simulink model "gm_Fixed"  (R2022a)
settings: Solver=FixedStepDiscrete  StartTime=0.0  StopTime=10.0  RelTol=1e-3  EnableMultiTasking=on
InitFcn:
  | test_init
settings Model: Creator=highi  LastModifiedBy=highi
settings OptimizationCC: BlockReduction=off  ConditionallyExecuteInputs=off
settings DebuggingCC: InheritedTsInSrcMsg=none
settings HardwareCC: ProdBitPerPointer=32  ProdBitPerSizeT=32  ProdBitPerPtrDiffT=32  ProdLargestAtomicFloat=None  ProdIntDivRoundTo=Undefined  ProdEndianess=Unspecified  ProdWordSize=32  ProdHWDeviceType=ASIC/FPGA->ASIC/FPGA  TargetBitPerPointer=64  TargetBitPerSizeT=64  TargetBitPerPtrDiffT=64  TargetLongLongMode=on  TargetIntDivRoundTo=Zero  TargetEndianess=LittleEndian  TargetWordSize=64  TargetHWDeviceType=Custom Processor->MATLAB Host Computer  ProdEqTarget=off

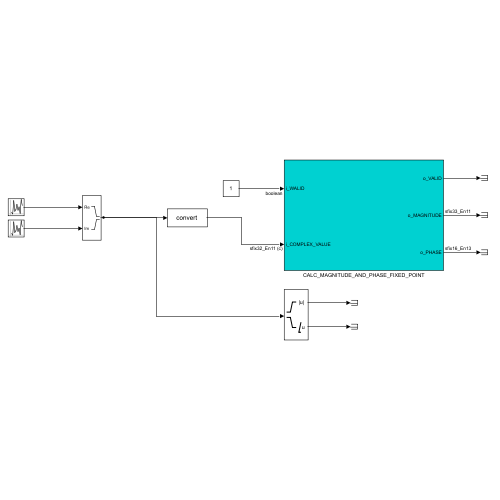
[thumbnail: Simulink's stored preview of the top-level diagram]
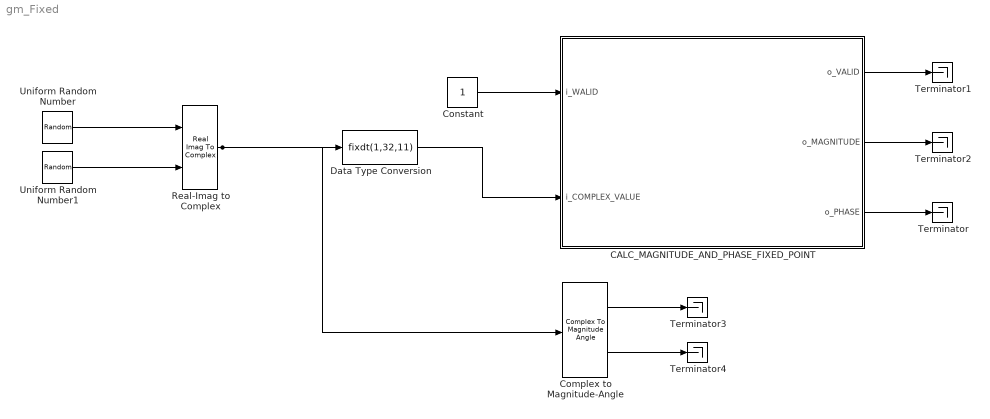
== system gm_Fixed ==
  CALC_MAGNITUDE_AND_PHASE_FIXED_POINT : Subsystem
  Complex to Magnitude-Angle : ComplexToMagnitudeAngle
  Constant : Constant  OutDataTypeStr=boolean  SampleTime=1
  Data Type Conversion : DataTypeConversion  OutDataTypeStr=fixdt(1,32,11)  RndMeth=Round
  Real-Imag to Complex : RealImagToComplex
  Terminator{,1..4} (5 alike) : Terminator
  Uniform Random Number : UniformRandomNumber  Minimum=0  Maximum=2097151.49999809265  Seed=21  SampleTime=1
  Uniform Random Number1 : UniformRandomNumber  Minimum=0  Maximum=2097151.49999809265  Seed=22  SampleTime=1
  wires:
  Complex to Magnitude-Angle/1 -> Terminator3/1
  Complex to Magnitude-Angle/2 -> Terminator4/1
  CALC_MAGNITUDE_AND_PHASE_FIXED_POINT/1(o_VALID) -> Terminator1/1
  CALC_MAGNITUDE_AND_PHASE_FIXED_POINT/2(o_MAGNITUDE) -> Terminator2/1
  CALC_MAGNITUDE_AND_PHASE_FIXED_POINT/3(o_PHASE) -> Terminator/1
  Constant/1 -> CALC_MAGNITUDE_AND_PHASE_FIXED_POINT/1(i_WALID)
  Data Type Conversion/1 -> CALC_MAGNITUDE_AND_PHASE_FIXED_POINT/2(i_COMPLEX_VALUE)
  Real-Imag to Complex/1 -> Data Type Conversion/1, Complex to Magnitude-Angle/1
  Uniform Random Number/1 -> Real-Imag to Complex/1
  Uniform Random Number1/1 -> Real-Imag to Complex/2

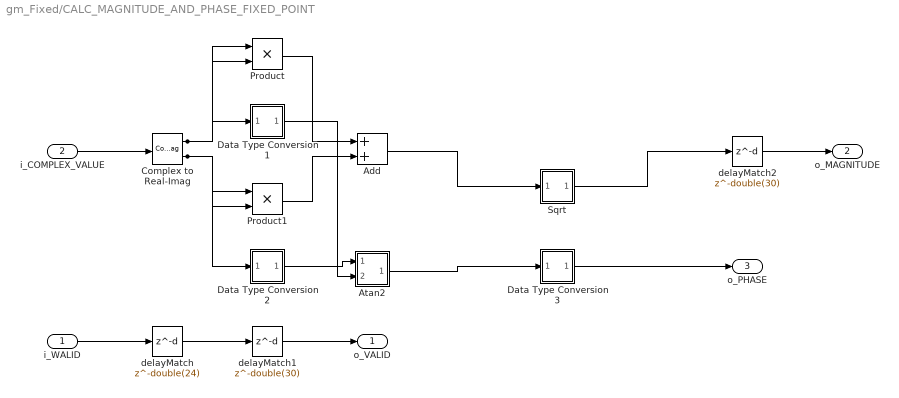
== system gm_Fixed/CALC_MAGNITUDE_AND_PHASE_FIXED_POINT ==
  i_WALID : Inport  OutDataTypeStr=boolean  PortDimensions=1  SampleTime=1
  i_COMPLEX_VALUE : Inport  Port=2  OutDataTypeStr=fixdt(1, 32, 11)  PortDimensions=1  SampleTime=1
      settings: SignalType=complex
  Add : Sum  AccumDataTypeStr=fixdt(1, 34, 11)  OutDataTypeStr=fixdt(1, 33, 11)  RndMeth=Round  SaturateOnIntegerOverflow=on  SampleTime=1
  Atan2 : Subsystem
      mask Display: disp('NFP\ntrig3');
  Complex to Real-Imag : ComplexToRealImag  SampleTime=1
  Data Type Conversion1 : Subsystem
      mask Display: disp('NFP\nconv');
  Data Type Conversion2 : Subsystem
      mask Display: disp('NFP\nconv');
  Data Type Conversion3 : Subsystem
      mask Display: disp('NFP\nconv');
  Product : Product  Inputs=**  OutDataTypeStr=fixdt(1, 33, 11)  RndMeth=Round  SaturateOnIntegerOverflow=on  SampleTime=1
  Product1 : Product  Inputs=**  OutDataTypeStr=fixdt(1, 33, 11)  RndMeth=Round  SaturateOnIntegerOverflow=on  SampleTime=1
  Sqrt : Subsystem
  delayMatch : Delay  DelayLength=double(24)  InitialCondition=0  SampleTime=1
  delayMatch1 : Delay  DelayLength=double(30)  InitialCondition=0  SampleTime=1
  delayMatch2 : Delay  DelayLength=double(30)  InitialCondition=0  SampleTime=1
  o_VALID : Outport  SampleTime=1
  o_MAGNITUDE : Outport  Port=2  OutDataTypeStr=fixdt(1,33,11)  SampleTime=1
  o_PHASE : Outport  Port=3  OutDataTypeStr=fixdt(1,16,13)  SampleTime=1
  wires:
  delayMatch1/1 -> o_VALID/1
  i_COMPLEX_VALUE/1 -> Complex to Real-Imag/1
  Add/1 -> Sqrt/1(In1)
  Complex to Real-Imag/1 -> Data Type Conversion1/1(In1), Product/2, Product/1
  Complex to Real-Imag/2 -> Data Type Conversion2/1(In1), Product1/2, Product1/1
  Product/1 -> Add/1
  Product1/1 -> Add/2
  delayMatch2/1 -> o_MAGNITUDE/1
  i_WALID/1 -> delayMatch/1
  Atan2/1(Out1) -> Data Type Conversion3/1(In1)
  Data Type Conversion1/1(Out1) -> Atan2/2(In2)
  Data Type Conversion2/1(Out1) -> Atan2/1(In1)
  Data Type Conversion3/1(Out1) -> o_PHASE/1
  delayMatch/1 -> delayMatch1/1
  Sqrt/1(Out1) -> delayMatch2/1

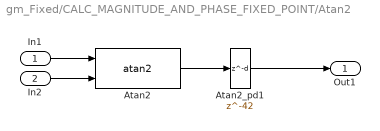
== system gm_Fixed/CALC_MAGNITUDE_AND_PHASE_FIXED_POINT/Atan2 ==
  In1 : Inport
  In2 : Inport  Port=2
  Atan2 : Trigonometry  Operator=atan2  SampleTime=1
  Atan2_pd1 : Delay  DelayLength=42
  Out1 : Outport
  wires:
  In1/1 -> Atan2/1
  In2/1 -> Atan2/2
  Atan2/1 -> Atan2_pd1/1
  Atan2_pd1/1 -> Out1/1

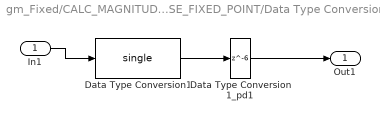
== system gm_Fixed/CALC_MAGNITUDE_AND_PHASE_FIXED_POINT/Data Type Conversion1 ==
  In1 : Inport
  Data Type Conversion1 : DataTypeConversion  OutDataTypeStr=single  SampleTime=1  SaturateOnIntegerOverflow=off  RndMeth=Floor
  Data Type Conversion1_pd1 : Delay  DelayLength=6
  Out1 : Outport
  wires:
  In1/1 -> Data Type Conversion1/1
  Data Type Conversion1/1 -> Data Type Conversion1_pd1/1
  Data Type Conversion1_pd1/1 -> Out1/1

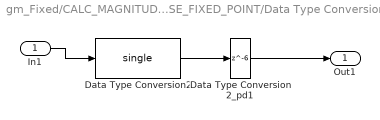
== system gm_Fixed/CALC_MAGNITUDE_AND_PHASE_FIXED_POINT/Data Type Conversion2 ==
  In1 : Inport
  Data Type Conversion2 : DataTypeConversion  OutDataTypeStr=single  SampleTime=1  SaturateOnIntegerOverflow=off  RndMeth=Floor
  Data Type Conversion2_pd1 : Delay  DelayLength=6
  Out1 : Outport
  wires:
  In1/1 -> Data Type Conversion2/1
  Data Type Conversion2/1 -> Data Type Conversion2_pd1/1
  Data Type Conversion2_pd1/1 -> Out1/1

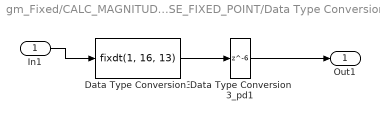
== system gm_Fixed/CALC_MAGNITUDE_AND_PHASE_FIXED_POINT/Data Type Conversion3 ==
  In1 : Inport
  Data Type Conversion3 : DataTypeConversion  OutDataTypeStr=fixdt(1, 16, 13)  RndMeth=Round  SampleTime=1  SaturateOnIntegerOverflow=off
  Data Type Conversion3_pd1 : Delay  DelayLength=6
  Out1 : Outport
  wires:
  In1/1 -> Data Type Conversion3/1
  Data Type Conversion3/1 -> Data Type Conversion3_pd1/1
  Data Type Conversion3_pd1/1 -> Out1/1

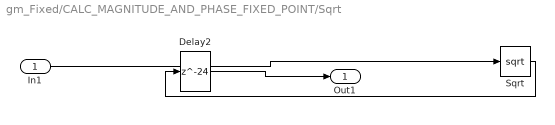
== system gm_Fixed/CALC_MAGNITUDE_AND_PHASE_FIXED_POINT/Sqrt ==
  In1 : Inport
  Delay2 : Delay  DelayLength=24
  Sqrt : Sqrt
  Out1 : Outport
  wires:
  In1/1 -> Sqrt/1
  Sqrt/1 -> Delay2/1
  Delay2/1 -> Out1/1
